simulink model "alpha147gta"  (R2016b)
settings: Solver=VariableStepAuto  StartTime=0.0  StopTime=10.0  RelTol=1e-3
PreLoadFcn:
  | load('alpha147gta.mat');
values from neighbouring files (symbols this model uses):
  EngineRPM = [1000 1500 2000 2500 3000 3500 4000 4500 5000 5500 6000 6500 ... (13 elements, 1x13)]    [alpha147gta.mat]
  EngineTRQ = [200 220 242 258 260 261 268 285 300 296 290 250 ... (13 elements, 1x13)]    [alpha147gta.mat]
  FinalRatio = 3.733    [alpha147gta.mat]
  GearRatio = [3.5 2.235 1.52 1.156 0.971 0.818]    [alpha147gta.mat]
  Kdrag = 0.4238432    [alpha147gta.mat]
  Mass = 1360    [alpha147gta.mat]
  WheelRadius = 0.2992    [alpha147gta.mat]
settings Model: Creator=bartb  LastModifiedBy=bartb

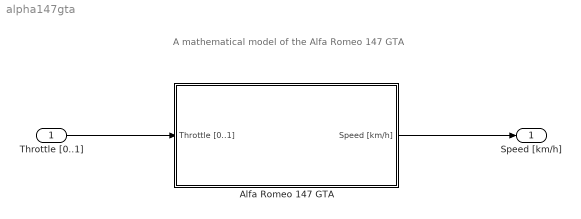
== system alpha147gta ==
  note: A mathematical model of the Alfa Romeo 147 GTA
  Throttle [0..1] : Inport
  Alfa Romeo 147 GTA : Subsystem
  Speed [km/h] : Outport
  wires:
  Throttle [0..1]/1 -> Alfa Romeo 147 GTA/1(Throttle [0..1])
  Alfa Romeo 147 GTA/1(Speed [km/h]) -> Speed [km/h]/1

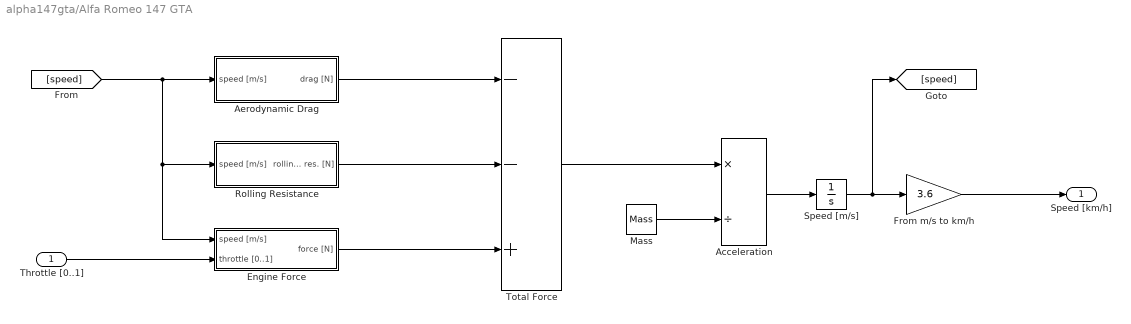
== system alpha147gta/Alfa Romeo 147 GTA ==
  Throttle [0..1] : Inport
  Acceleration : Product  Inputs=*/
  Aerodynamic Drag : Subsystem
  Engine Force : Subsystem
  From m/s to km/h : Gain  Gain=3.6
  Mass : Constant  Value=Mass
  Rolling Resistance : Subsystem
  Speed [m/s] : Integrator
  Total Force : Sum  Inputs=--+
  Speed [km/h] : Outport
  wires:
  Throttle [0..1]/1 -> Engine Force/2(throttle [0..1])
  Engine Force/1(force [N]) -> Total Force/3
  Rolling Resistance/1(rolling res. [N]) -> Total Force/2
  Aerodynamic Drag/1(drag [N]) -> Total Force/1
  Mass/1 -> Acceleration/2
  Total Force/1 -> Acceleration/1
  Acceleration/1 -> Speed [m/s]/1
  Speed [m/s]/1 -> [speed], From m/s to km/h/1
  From m/s to km/h/1 -> Speed [km/h]/1
  [speed] -> Engine Force/1(speed [m/s]), Rolling Resistance/1(speed [m/s]), Aerodynamic Drag/1(speed [m/s])

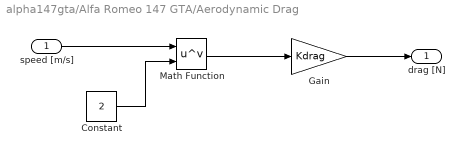
== system alpha147gta/Alfa Romeo 147 GTA/Aerodynamic Drag ==
  speed [m/s] : Inport
  Constant : Constant  Value=2
  Gain : Gain  Gain=Kdrag
  Math Function : Math  Operator=pow  SaturateOnIntegerOverflow=on
  drag [N] : Outport
  wires:
  speed [m/s]/1 -> Math Function/1
  Constant/1 -> Math Function/2
  Math Function/1 -> Gain/1
  Gain/1 -> drag [N]/1

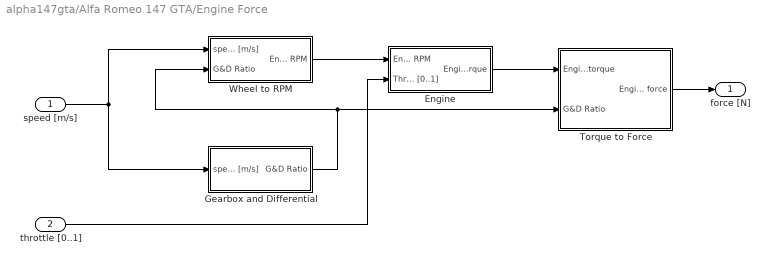
== system alpha147gta/Alfa Romeo 147 GTA/Engine Force ==
  speed [m/s] : Inport
  throttle [0..1] : Inport  Port=2
  Engine : Subsystem
  Gearbox and Differential : Subsystem
  Torque to Force : Subsystem
  Wheel to RPM : Subsystem
  force [N] : Outport
  wires:
  Wheel to RPM/1(Engine RPM) -> Engine/1(Engine RPM)
  speed [m/s]/1 -> Gearbox and Differential/1(speed [m/s]), Wheel to RPM/1(speed [m/s])
  Gearbox and Differential/1(G&D Ratio) -> Wheel to RPM/2(G&D Ratio), Torque to Force/2(G&D Ratio)
  throttle [0..1]/1 -> Engine/2(Throttle [0..1])
  Engine/1(Engine Torque) -> Torque to Force/1(Engine torque)
  Torque to Force/1(Engine force) -> force [N]/1

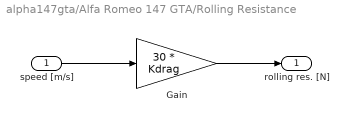
== system alpha147gta/Alfa Romeo 147 GTA/Rolling Resistance ==
  speed [m/s] : Inport
  Gain : Gain  Gain=30 * Kdrag
  rolling res. [N] : Outport
  wires:
  speed [m/s]/1 -> Gain/1
  Gain/1 -> rolling res. [N]/1

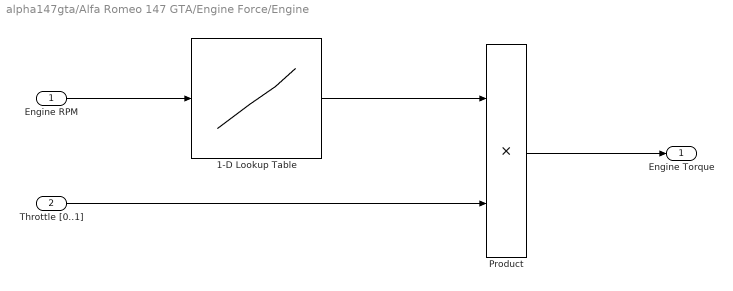
== system alpha147gta/Alfa Romeo 147 GTA/Engine Force/Engine ==
  Engine RPM : Inport
  Throttle [0..1] : Inport  Port=2
  1-D Lookup Table : Lookup_n-D  NumberOfTableDimensions=1  BreakpointsForDimension1=EngineRPM  Table=EngineTRQ  InterpMethod=Cubic spline  InternalRulePriority=Speed  RndMeth=Simplest  InputSameDT=on
  Product : Product
  Engine Torque : Outport
  wires:
  Engine RPM/1 -> 1-D Lookup Table/1
  1-D Lookup Table/1 -> Product/1
  Throttle [0..1]/1 -> Product/2
  Product/1 -> Engine Torque/1

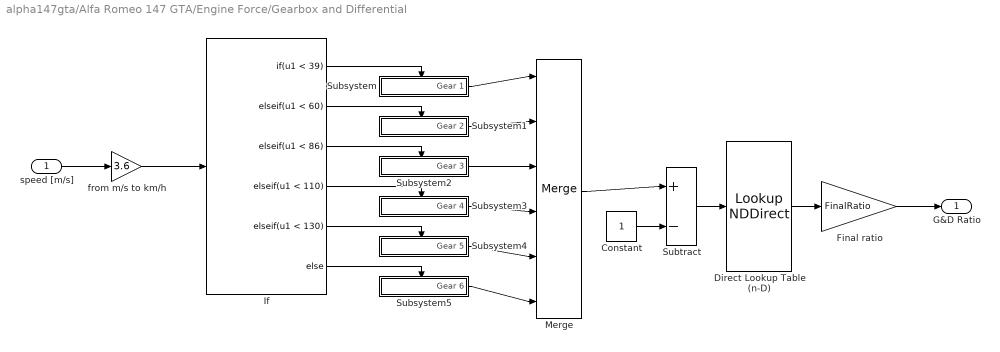
== system alpha147gta/Alfa Romeo 147 GTA/Engine Force/Gearbox and Differential ==
  speed [m/s] : Inport
  " Subsystem" : Subsystem  TreatAsAtomicUnit=on
  " Subsystem1" : Subsystem  TreatAsAtomicUnit=on
  " Subsystem2" : Subsystem  TreatAsAtomicUnit=on
  " Subsystem3" : Subsystem  TreatAsAtomicUnit=on
  " Subsystem4" : Subsystem  TreatAsAtomicUnit=on
  " Subsystem5" : Subsystem  TreatAsAtomicUnit=on
  Constant : Constant
  Direct Lookup Table (n-D) : LookupNDDirect  NumberOfTableDimensions=1  Table=GearRatio
  Final ratio : Gain  Gain=FinalRatio
  If : If  IfExpression=u1 < 39  ElseIfExpressions=u1 < 60, u1 < 86, u1 < 110, u1 < 130
  Merge : Merge  Inputs=6
  Subtract : Sum  Inputs=+-
  from m/s to km/h : Gain  Gain=3.6
  G&D Ratio : Outport
  wires:
  speed [m/s]/1 -> from m/s to km/h/1
  from m/s to km/h/1 -> If/1
  If/2 -> " Subsystem1"/Action
  If/3 -> " Subsystem2"/Action
  If/4 -> " Subsystem3"/Action
  If/5 -> " Subsystem4"/Action
  If/6 -> " Subsystem5"/Action
  If/1 -> " Subsystem"/Action
  " Subsystem"/1(Gear 1) -> Merge/1
  " Subsystem1"/1(Gear 2) -> Merge/2
  " Subsystem2"/1(Gear 3) -> Merge/3
  " Subsystem3"/1(Gear 4) -> Merge/4
  " Subsystem4"/1(Gear 5) -> Merge/5
  " Subsystem5"/1(Gear 6) -> Merge/6
  Constant/1 -> Subtract/2
  Merge/1 -> Subtract/1
  Subtract/1 -> Direct Lookup Table (n-D)/1
  Direct Lookup Table (n-D)/1 -> Final ratio/1
  Final ratio/1 -> G&D Ratio/1

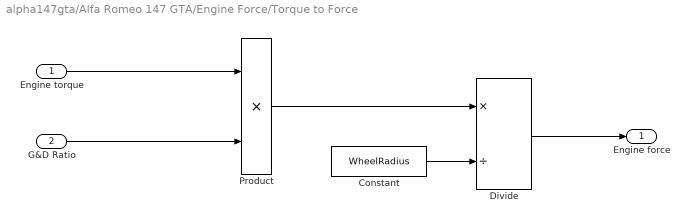
== system alpha147gta/Alfa Romeo 147 GTA/Engine Force/Torque to Force ==
  Engine torque : Inport
  G&D Ratio : Inport  Port=2
  Constant : Constant  Value=WheelRadius
  Divide : Product  Inputs=*/
  Product : Product
  Engine force : Outport
  wires:
  Engine torque/1 -> Product/1
  G&D Ratio/1 -> Product/2
  Constant/1 -> Divide/2
  Product/1 -> Divide/1
  Divide/1 -> Engine force/1

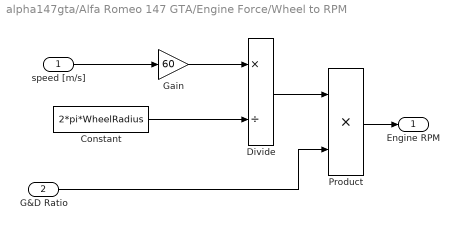
== system alpha147gta/Alfa Romeo 147 GTA/Engine Force/Wheel to RPM ==
  speed [m/s] : Inport
  G&D Ratio : Inport  Port=2
  Constant : Constant  Value=2*pi*WheelRadius
  Divide : Product  Inputs=*/
  Gain : Gain  Gain=60
  Product : Product
  Engine RPM : Outport
  wires:
  speed [m/s]/1 -> Gain/1
  Constant/1 -> Divide/2
  Gain/1 -> Divide/1
  Divide/1 -> Product/1
  G&D Ratio/1 -> Product/2
  Product/1 -> Engine RPM/1

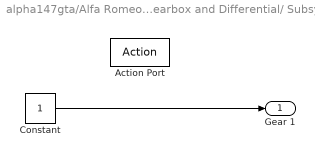
== system alpha147gta/Alfa Romeo 147 GTA/Engine Force/Gearbox and Differential/ Subsystem ==
  Action Port : ActionPort  ActionType=then
  Constant : Constant
  Gear 1 : Outport
  wires:
  Constant/1 -> Gear 1/1

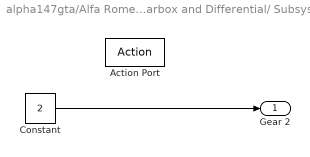
== system alpha147gta/Alfa Romeo 147 GTA/Engine Force/Gearbox and Differential/ Subsystem1 ==
  Action Port : ActionPort  ActionType=elseif
  Constant : Constant  Value=2
  Gear 2 : Outport
  wires:
  Constant/1 -> Gear 2/1

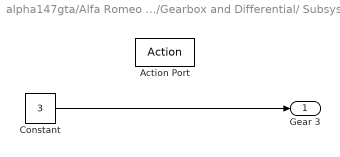
== system alpha147gta/Alfa Romeo 147 GTA/Engine Force/Gearbox and Differential/ Subsystem2 ==
  Action Port : ActionPort  ActionType=elseif
  Constant : Constant  Value=3
  Gear 3 : Outport
  wires:
  Constant/1 -> Gear 3/1

== system alpha147gta/Alfa Romeo 147 GTA/Engine Force/Gearbox and Differential/ Subsystem3 ==
  Action Port : ActionPort  ActionType=elseif
  Constant : Constant  Value=4
  Gear 4 : Outport
  wires:
  Constant/1 -> Gear 4/1

== system alpha147gta/Alfa Romeo 147 GTA/Engine Force/Gearbox and Differential/ Subsystem4 ==
  Action Port : ActionPort  ActionType=elseif
  Constant : Constant  Value=5
  Gear 5 : Outport
  wires:
  Constant/1 -> Gear 5/1

== system alpha147gta/Alfa Romeo 147 GTA/Engine Force/Gearbox and Differential/ Subsystem5 ==
  Action Port : ActionPort  ActionType=else
  Constant : Constant  Value=6
  Gear 6 : Outport
  wires:
  Constant/1 -> Gear 6/1
